simulink model "myfuzzyPID"  (R2014a)
settings: Solver=ode45  StartTime=0.0  StopTime=10.0  RelTol=1e-3
values from neighbouring files (symbols this model uses):
  matrix = readfis('fuzzyPID.fis')    [fuzzy.m]
libraries: fuzblock x1
settings Model: Creator=Administrator  LastModifiedBy=Administrator

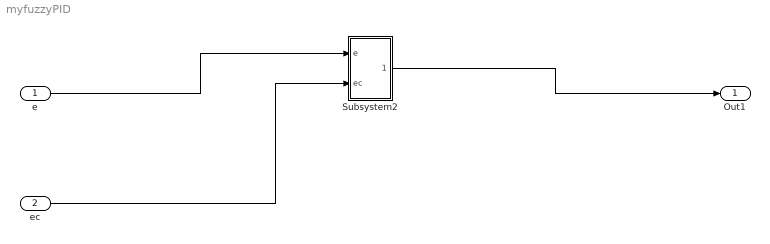
== system myfuzzyPID ==
  e : Inport
  ec : Inport  Port=2
  Subsystem2 : Subsystem
  Out1 : Outport
  wires:
  e/1 -> Subsystem2/1(e)
  ec/1 -> Subsystem2/2(ec)
  Subsystem2/1(Out1) -> Out1/1

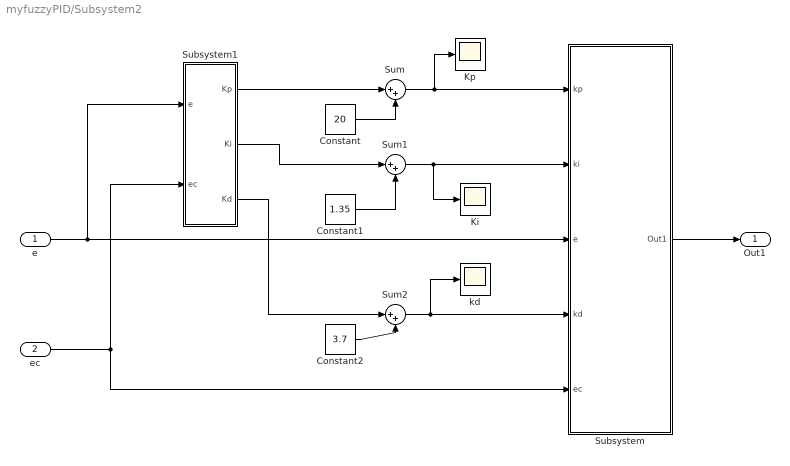
== system myfuzzyPID/Subsystem2 ==
  e : Inport
  ec : Inport  Port=2
  Constant : Constant  Value=20
  Constant1 : Constant  Value=1.35
  Constant2 : Constant  Value=3.7
  Ki : Scope
  Kp : Scope
  Subsystem : Subsystem
  Subsystem1 : Subsystem
  Sum : Sum  Inputs=|++
  Sum1 : Sum  Inputs=|++
  Sum2 : Sum  Inputs=|++
  kd : Scope
      settings: SaveName=ScopeData2
  Out1 : Outport
  wires:
  Sum2/1 -> kd/1, Subsystem/4(kd)
  Constant/1 -> Sum/2
  Subsystem1/1(Kp) -> Sum/1
  Subsystem1/2(Ki) -> Sum1/1
  e/1 -> Subsystem/3(e), Subsystem1/1(e)
  Subsystem/1(Out1) -> Out1/1
  Sum/1 -> Kp/1, Subsystem/1(kp)
  ec/1 -> Subsystem1/2(ec), Subsystem/5(ec)
  Constant2/1 -> Sum2/2
  Constant1/1 -> Sum1/2
  Subsystem1/3(Kd) -> Sum2/1
  Sum1/1 -> Ki/1, Subsystem/2(ki)

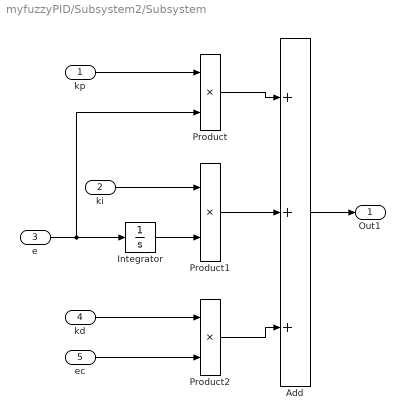
== system myfuzzyPID/Subsystem2/Subsystem ==
  kp : Inport
  ki : Inport  Port=2
  e : Inport  Port=3
  kd : Inport  Port=4
  ec : Inport  Port=5
  Add : Sum  Inputs=+++
  Integrator : Integrator
  Product : Product
  Product1 : Product
  Product2 : Product
  Out1 : Outport
  wires:
  kd/1 -> Product2/1
  Integrator/1 -> Product1/2
  e/1 -> Product/2, Integrator/1
  ec/1 -> Product2/2
  Product/1 -> Add/1
  Product1/1 -> Add/2
  Product2/1 -> Add/3
  Add/1 -> Out1/1
  ki/1 -> Product1/1
  kp/1 -> Product/1

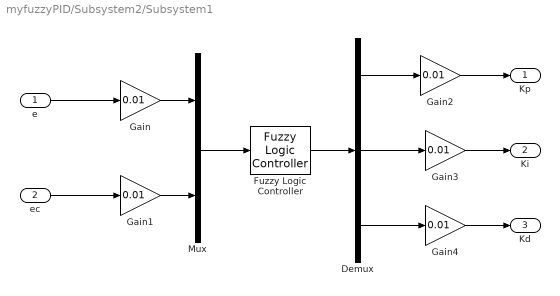
== system myfuzzyPID/Subsystem2/Subsystem1 ==
  e : Inport
  ec : Inport  Port=2
  Demux : Demux  Outputs=3
  Fuzzy Logic Controller : fuzblock/Fuzzy Logic  Controller  fis=[matrix]
  Gain{,1..4} (5 alike) : Gain  Gain=0.01
  Mux : Mux  Inputs=2
  Kp : Outport
  Ki : Outport  Port=2
  Kd : Outport  Port=3
  wires:
  e/1 -> Gain/1
  Gain1/1 -> Mux/2
  Gain/1 -> Mux/1
  ec/1 -> Gain1/1
  Fuzzy Logic Controller/1 -> Demux/1
  Gain4/1 -> Kd/1
  Gain2/1 -> Kp/1
  Mux/1 -> Fuzzy Logic Controller/1
  Gain3/1 -> Ki/1
  Demux/2 -> Gain3/1
  Demux/1 -> Gain2/1
  Demux/3 -> Gain4/1
